simulink model "NXPFRDMK64F"  (R2022a)
settings: Solver=FixedStepAuto  StartTime=0.0  StopTime=60  FixedStep=1e-3  RelTol=1e-3  EnableMultiTasking=on
undefined symbols (not defined in the file): A0, A1, ARPtest, ATRsense, D0, D1, D10, D11, D12, D13, D2, D3, D4, D5, D6, D7, D8, D9, LRLtest, PTA0, PTA1, PTA2, PTB2, PTB23, PTB3, PTB9, PTC16, PTC17, PTC2, PTC3, PTC4, PTD0, PTD1, PTD2, PTD3, pulsewtest, URLtest, VENTsense, VRPtest
libraries: frdmk64flib x20, simulink x2, etargetslib x2
settings Model: ExtModeTrigDuration=5  Creator=patri  LastModifiedBy=David
settings OptimizationCC: EnhancedBackFolding=on  PassReuseOutputArgsAs=Individual arguments  ZeroExternalMemoryAtStartup=off  ZeroInternalMemoryAtStartup=off  MaxStackSize=64  OptimizeBlockOrder=speed  DifferentSizesBufferReuse=on  OptimizationCustomize=off  EfficientTunableParamExpr=on
settings DebuggingCC: ParameterTunabilityLossMsg=error
settings HardwareCC: ProdBitPerPointer=32  ProdBitPerSizeT=32  ProdBitPerPtrDiffT=32  ProdLargestAtomicInteger=Long  ProdLargestAtomicFloat=Double  ProdWordSize=32  ProdHWDeviceType=ARM Compatible->ARM Cortex
settings SFSimCC: MATLABDynamicMemAlloc=off
settings RTWCC: SystemTargetFile=ert.tlc  HardwareBoard=NXP FRDM-K64F  TLCOptions="-aInlineSetEventsForThisBaseRateFcn=TLC_FALSE -aSuppressMultiTaskScheduler=TLC_FALSE  -aRateBasedStepFcn=0"  TemplateMakefile=ert_default_tmf  Toolchain=GNU Tools for ARM Embedded Processors
settings CodeAppCC: ForceParamTrailComments=on  IgnoreCustomStorageClasses=off  OperatorAnnotations=on  SimulinkDataObjDesc=on  SFDataObjDesc=on  InsertBlockDesc=on
settings ERTTargetCC: ExtModeTransport=4  ExtModeMexFile=sendToCommService

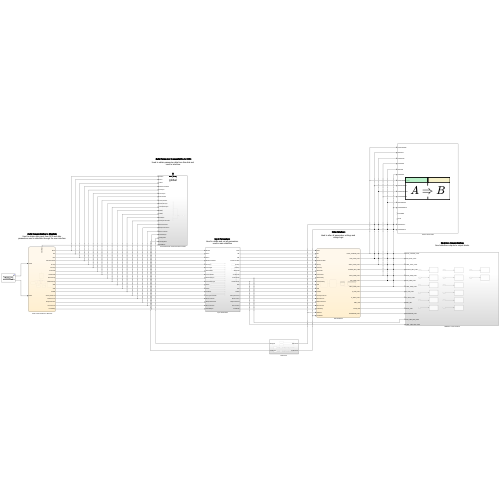
[thumbnail: Simulink's stored preview of the top-level diagram]
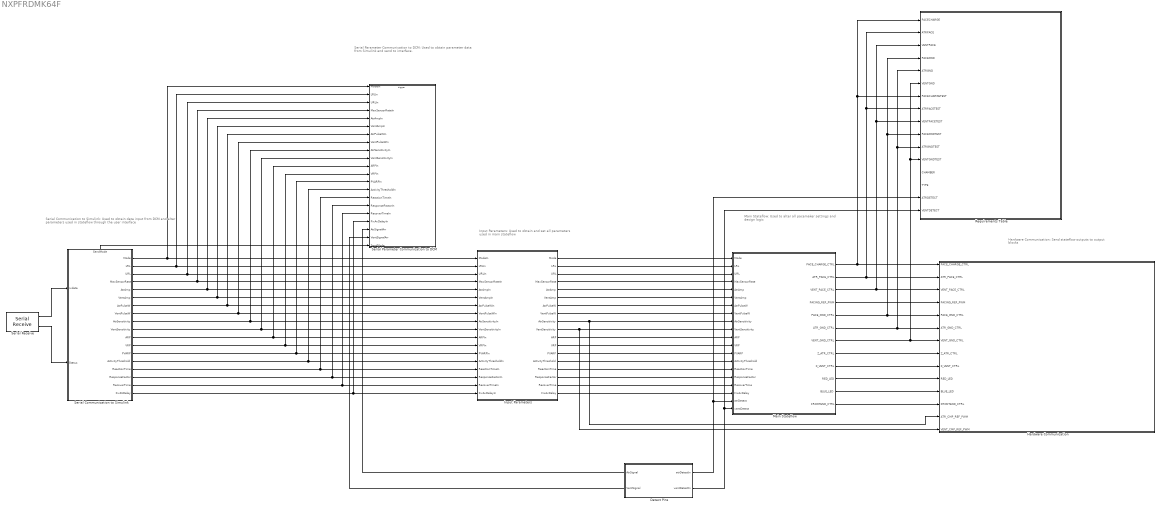
== system NXPFRDMK64F ==
  note: Input Parameters:
      | Used to obtain and set all parameters
      | used in main stateflow
  note: Main Stateflow:
      | Used to alter all pacemaker settings and
      | design logic
  note: Hardware Communication:
      | Send stateflow outputs to output blocks
  note: Serial Communication to Simulink:
      | Used to obtain data input from DCM and alter
      | parameters used in stateflow through the user interface
  note: Serial Parameter Communication to DCM:
      | Used to obtain parameter data from Simulink and
      | send to interface.
  Detect Pins : Subsystem
      settings: PortSchema="{\"entries\":[{\"content\":{\"sides\":[{\"content\":{\"connectorIds\":[\"Out3\",\"Out4\"]},\"type\":\"ConnectorPlacement.EquallySpacedRectSide\",\"uuid\":\"22ae5160-7907-4e02-9170-83912aa0621b\"},{\"content\":{\"connectorIds\":[\"Out1\",\"Out2\"],\"side\":\"RIGHT\"},\"type\":\"ConnectorPlacement.EquallySpacedRectSide\",\"uuid\":\"4a288593-63c5-4fb6-8cc6-6c5672326909\"},{\"content\":{\"connectorIds\":[],\"side\":\"TOP\"},\"type\":\"ConnectorPlacement.EquallySpacedRectSide\",\"uuid\":\"225d709c-1657-4037-9f08-1b7c425ad473\"}]},\"type\":\"ConnectorPlacement.EquallySpacedConnector\",\"uuid\":\"4f29d97d-bf7f-4e6d-a194-73bc61128bb5\"}],\"packageUris\":[\"http://schema.mathworks.com/mf0/Connector/R2020b\"],\"version\":\"1.0\"}"
  Hardware Communication : Subsystem
  Input Parameters : Subsystem
  Main Stateflow : Stateflow chart  TreatAsAtomicUnit=on
  Requirements Table : Requirements Table  TreatAsAtomicUnit=on
  Serial Communication to Simulink : Stateflow chart  TreatAsAtomicUnit=on
      settings: PortSchema="{\"entries\":[{\"content\":{\"sides\":[{\"content\":{\"connectorIds\":[\"In1\",\"In2\"]},\"type\":\"ConnectorPlacement.EquallySpacedRectSide\",\"uuid\":\"59d5f214-816c-4a61-90ca-5ecc2aac6342\"},{\"content\":{\"connectorIds\":[\"Out1\",\"Out2\",\"Out3\",\"Out4\",\"Out5\",\"Out6\",\"Out7\",\"Out8\",\"Out9\",\"Out10\",\"Out11\",\"Out12\",\"Out13\",\"Out14\",\"Out15\",\"Out16\",\"Out17\",\"Out18\"],\"side\":\"RIGHT\"},\"type\":\"ConnectorPlacement.EquallySpacedRectSide\",\"uuid\":\"caa3dc8d-9426-4e4b-b542-59ffb9e9ff55\"},{\"content\":{\"connectorIds\":[\"Out19\"],\"side\":\"TOP\"},\"type\":\"ConnectorPlacement.EquallySpacedRectSide\",\"uuid\":\"7c0b9c62-6555-43d5-acbe-ad9d7bd12e4a\"}]},\"type\":\"ConnectorPlacement.EquallySpacedConnector\",\"uuid\":\"af3c612b-0d58-4e05-b024-fac367dc3217\"}],\"packageUris\":[\"http://schema.mathworks.com/mf0/Connector/R2020b\"],\"version\":\"1.0\"}"
  Serial Parameter Communication to DCM : Subsystem  TreatAsAtomicUnit=on
  Serial Receive : frdmk64flib/Serial Receive  SCIModule=0  Baudrate=uint32(9600)  Parity=None  StopBits=1  HardwareFlowControl=None  ByteOrder=LittleEndian  DataType=uint8  DataLength=20  BlockingMode=off  OutputStatus=on  SampleTime=-1
  wires:
  Main Stateflow/1(PACE_CHARGE_CTRL) -> Requirements Table/1(PACECHARGE), Requirements Table/7(PACECHARGETEST), Hardware Communication/1(PACE_CHARGE_CTRL)
  Main Stateflow/3(VENT_PACE_CTRL) -> Requirements Table/3(VENTPACE), Requirements Table/9(VENTPACETEST), Hardware Communication/3(VENT_PACE_CTRL)
  Main Stateflow/4(PACING_REF_PWM) -> Hardware Communication/4(PACING_REF_PWM)
  Main Stateflow/5(PACE_GND_CTRL) -> Requirements Table/4(PACEGND), Requirements Table/10(PACEGNDTEST), Hardware Communication/5(PACE_GND_CTRL)
  Main Stateflow/8(Z_ATR_CTRL) -> Hardware Communication/8("Z_ATR_CTRL ")
  Main Stateflow/9(Z_VENT_CTRL) -> Hardware Communication/9(Z_VENT_CTRL)
  Main Stateflow/11(BLUE_LED) -> Hardware Communication/11(BLUE_LED)
  Main Stateflow/10(RED_LED) -> Hardware Communication/10(RED_LED)
  Main Stateflow/6(ATR_GND_CTRL) -> Requirements Table/5(ATRGND), Requirements Table/11(ATRGNDTEST), Hardware Communication/6(ATR_GND_CTRL)
  Main Stateflow/2(ATR_PACE_CTRL) -> Requirements Table/2(ATRPACE), Requirements Table/8(ATRPACETEST), Hardware Communication/2(ATR_PACE_CTRL)
  Main Stateflow/12(FRONTEND_CTRL) -> Hardware Communication/12(FRONTEND_CTRL)
  Detect Pins/2(ventDetectIn) -> Requirements Table/16(VENTDETECT), Main Stateflow/20(ventDetect)
  Serial Receive/1 -> Serial Communication to Simulink/1(rxdata)
  Serial Receive/2 -> Serial Communication to Simulink/2(Status)
  Main Stateflow/7(VENT_GND_CTRL) -> Requirements Table/6(VENTGND), Requirements Table/12(VENTGNDTEST), Hardware Communication/7(VENT_GND_CTRL)
  Detect Pins/1(atrDetectIn) -> Requirements Table/15(ATRDETECT), Main Stateflow/19(atrDetect)
  Serial Communication to Simulink/1(Mode) -> Serial Parameter Communication to DCM/1(ModeIn), Input Parameters/1(ModeIn)
  Serial Communication to Simulink/2(LRL) -> Serial Parameter Communication to DCM/2(LRLIn), Input Parameters/2(LRLIn)
  Serial Communication to Simulink/3(URL) -> Serial Parameter Communication to DCM/3(URLIn), Input Parameters/3(URLIn)
  Serial Communication to Simulink/4(MaxSensorRate) -> Serial Parameter Communication to DCM/4(MaxSensorRateIn), Input Parameters/4(MaxSensorRateIn)
  Serial Communication to Simulink/5(AtrAmp) -> Serial Parameter Communication to DCM/5(AtrAmpIn), Input Parameters/5(AtrAmpIn)
  Serial Communication to Simulink/7(AtrPulseW) -> Serial Parameter Communication to DCM/7(AtrPulseWIn), Input Parameters/7(AtrPulseWIn)
  Serial Communication to Simulink/6(VentAmp) -> Serial Parameter Communication to DCM/6(VentAmpIn), Input Parameters/6(VentAmpIn)
  Serial Communication to Simulink/8(VentPulseW) -> Serial Parameter Communication to DCM/8(VentPulseWIn), Input Parameters/8(VentPulseWIn)
  Serial Communication to Simulink/10(VentSensitivity) -> Serial Parameter Communication to DCM/10(VentSensitivityIn), Input Parameters/10(VentSensitivityIn)
  Serial Communication to Simulink/11(ARP) -> Serial Parameter Communication to DCM/11(ARPIn), Input Parameters/11(ARPIn)
  Serial Communication to Simulink/9(AtrSensitivity) -> Serial Parameter Communication to DCM/9(AtrSensitivityIn), Input Parameters/9(AtrSensitivityIn)
  Serial Communication to Simulink/12(VRP) -> Serial Parameter Communication to DCM/12(VRPIn), Input Parameters/12(VRPIn)
  Serial Communication to Simulink/13(PVARP) -> Serial Parameter Communication to DCM/13(PVARPIn), Input Parameters/13(PVARPIn)
  Serial Communication to Simulink/14(ActivityThreshold) -> Serial Parameter Communication to DCM/14(ActivityThresholdIn), Input Parameters/14(ActivityThresholdIn)
  Serial Communication to Simulink/15(ReactionTime) -> Serial Parameter Communication to DCM/15(ReactionTimeIn), Input Parameters/15(ReactionTimeIn)
  Serial Communication to Simulink/16(ResponseFactor) -> Serial Parameter Communication to DCM/16(ResponseFactorIn), Input Parameters/16(ResponseFactorIn)
  Serial Communication to Simulink/17(RecoverTime) -> Serial Parameter Communication to DCM/17(RecoverTimeIn), Input Parameters/17(RecoverTimeIn)
  Serial Communication to Simulink/18(FixAVDelay) -> Serial Parameter Communication to DCM/18(FixAvDelayIn), Input Parameters/18(FixAvDelayIn)
  Detect Pins/4(VentSignal) -> Serial Parameter Communication to DCM/20(VentSignalArr)
  Detect Pins/3(AtrSignal) -> Serial Parameter Communication to DCM/19(AtrSignalArr)
  Input Parameters/1(Mode) -> Main Stateflow/1(Mode)
  Input Parameters/2(LRL) -> Main Stateflow/2(LRL)
  Input Parameters/3(URL) -> Main Stateflow/3(URL)
  Input Parameters/4(MaxSensorRate) -> Main Stateflow/4(MaxSensorRate)
  Input Parameters/5(AtrAmp) -> Main Stateflow/5(AtrAmp)
  Input Parameters/6(VentAmp) -> Main Stateflow/6(VentAmp)
  Input Parameters/7(AtrPulseW) -> Main Stateflow/7(AtrPulseW)
  Input Parameters/8(VentPulseW) -> Main Stateflow/8(VentPulseW)
  Input Parameters/9(AtrSensitivity) -> Hardware Communication/13(ATR_CMP_REF_PWM), Main Stateflow/9(AtrSensitivity)
  Input Parameters/10(VentSensitivity) -> Hardware Communication/14(VENT_CMP_REF_PWM), Main Stateflow/10(VentSensitivity)
  Input Parameters/11(ARP) -> Main Stateflow/11(ARP)
  Input Parameters/14(ActivityThreshold) -> Main Stateflow/14(ActivityThreshold)
  Input Parameters/13(PVARP) -> Main Stateflow/13(PVARP)
  Input Parameters/12(VRP) -> Main Stateflow/12(VRP)
  Input Parameters/15(ReactionTime) -> Main Stateflow/15(ReactionTime)
  Input Parameters/16(ResponseFactor) -> Main Stateflow/16(ResponseFactor)
  Input Parameters/17(RecoverTime) -> Main Stateflow/17(RecoverTime)
  Input Parameters/18(FixAvDelay) -> Main Stateflow/18(FixAvDelay)
  Serial Communication to Simulink/19(SendMode) -> Serial Parameter Communication to DCM/21(SendMode)

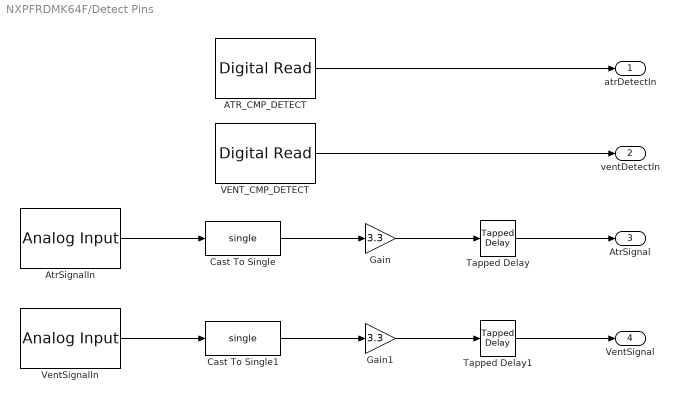
== system NXPFRDMK64F/Detect Pins ==
  ATR_CMP_DETECT : frdmk64flib/Digital Read  Whichpin=PTC16 (D0)  SampleTime=-1
  AtrSignalIn : frdmk64flib/Analog Input  Whichpin=PTB2 (A0)  SampleTime=-1
  Cast To Single : DataTypeConversion  OutDataTypeStr=single  SaturateOnIntegerOverflow=off  RndMeth=Floor
  Cast To Single1 : DataTypeConversion  OutDataTypeStr=single  SaturateOnIntegerOverflow=off  RndMeth=Floor
  Gain : Gain  Gain=3.3
  Gain1 : Gain  Gain=3.3
  Tapped Delay : simulink/Discrete/Tapped Delay  vinit=0.0  samptime=0.002  NumDelays=9  DelayOrder=Oldest  includeCurrent=off
  Tapped Delay1 : simulink/Discrete/Tapped Delay  vinit=0.0  samptime=0.002  NumDelays=9  DelayOrder=Oldest  includeCurrent=off
  VENT_CMP_DETECT : frdmk64flib/Digital Read  Whichpin=PTC17 (D1)  SampleTime=-1
  VentSignalIn : frdmk64flib/Analog Input  Whichpin=PTB3 (A1)  SampleTime=-1
  atrDetectIn : Outport
  ventDetectIn : Outport  Port=2
  AtrSignal : Outport  Port=3
  VentSignal : Outport  Port=4
  wires:
  VENT_CMP_DETECT/1 -> ventDetectIn/1
  ATR_CMP_DETECT/1 -> atrDetectIn/1
  AtrSignalIn/1 -> Cast To Single/1
  Cast To Single/1 -> Gain/1
  Gain/1 -> Tapped Delay/1
  Tapped Delay/1 -> AtrSignal/1
  Gain1/1 -> Tapped Delay1/1
  Cast To Single1/1 -> Gain1/1
  Tapped Delay1/1 -> VentSignal/1
  VentSignalIn/1 -> Cast To Single1/1

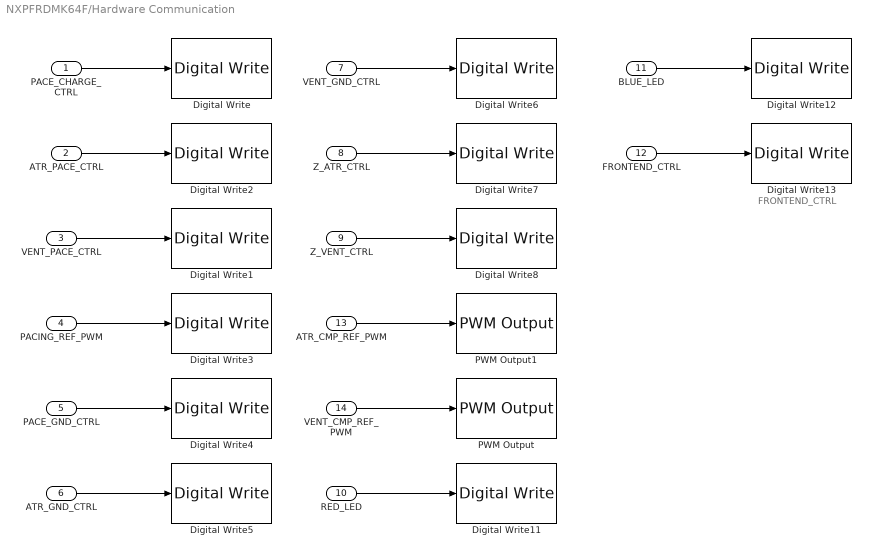
== system NXPFRDMK64F/Hardware Communication ==
  note: FRONTEND_CTRL
  PACE_CHARGE_CTRL : Inport
  ATR_PACE_CTRL : Inport  Port=2
  VENT_PACE_CTRL : Inport  Port=3
  PACING_REF_PWM : Inport  Port=4
  PACE_GND_CTRL : Inport  Port=5
  ATR_GND_CTRL : Inport  Port=6
  VENT_GND_CTRL : Inport  Port=7
  "Z_ATR_CTRL " : Inport  Port=8
  Z_VENT_CTRL : Inport  Port=9
  RED_LED : Inport  Port=10
  BLUE_LED : Inport  Port=11
  FRONTEND_CTRL : Inport  Port=12
  ATR_CMP_REF_PWM : Inport  Port=13
  VENT_CMP_REF_PWM : Inport  Port=14
  Digital Write : frdmk64flib/Digital Write  Whichpin=PTB9 (D2)
  Digital Write1 : frdmk64flib/Digital Write  Whichpin=PTC4 (D9)
  Digital Write11 : frdmk64flib/Digital Write  Whichpin=RED_LED
  Digital Write12 : frdmk64flib/Digital Write  Whichpin=BLUE_LED
  Digital Write13 : frdmk64flib/Digital Write  Whichpin=PTD1 (D13)
  Digital Write2 : frdmk64flib/Digital Write  Whichpin=PTA0 (D8)
  Digital Write3 : frdmk64flib/Digital Write  Whichpin=PTA2 (D5)
  Digital Write4 : frdmk64flib/Digital Write  Whichpin=PTD0 (D10)
  Digital Write5 : frdmk64flib/Digital Write  Whichpin=PTD2 (D11)
  Digital Write6 : frdmk64flib/Digital Write  Whichpin=PTD3 (D12)
  Digital Write7 : frdmk64flib/Digital Write  Whichpin=PTB23 (D4)
  Digital Write8 : frdmk64flib/Digital Write  Whichpin=PTC3 (D7)
  PWM Output : frdmk64flib/PWM Output  Whichpin=PTA1 (D3)  InitialFrequency=2000  InitialDutyCycle=0
  PWM Output1 : frdmk64flib/PWM Output  Whichpin=PTC2 (D6)  InitialFrequency=2000  InitialDutyCycle=0
  wires:
  "Z_ATR_CTRL "/1 -> Digital Write7/1
  ATR_CMP_REF_PWM/1 -> PWM Output1/1
  Z_VENT_CTRL/1 -> Digital Write8/1
  VENT_CMP_REF_PWM/1 -> PWM Output/1
  BLUE_LED/1 -> Digital Write12/1
  PACE_CHARGE_CTRL/1 -> Digital Write/1
  RED_LED/1 -> Digital Write11/1
  ATR_PACE_CTRL/1 -> Digital Write2/1
  VENT_PACE_CTRL/1 -> Digital Write1/1
  PACING_REF_PWM/1 -> Digital Write3/1
  PACE_GND_CTRL/1 -> Digital Write4/1
  ATR_GND_CTRL/1 -> Digital Write5/1
  VENT_GND_CTRL/1 -> Digital Write6/1
  FRONTEND_CTRL/1 -> Digital Write13/1

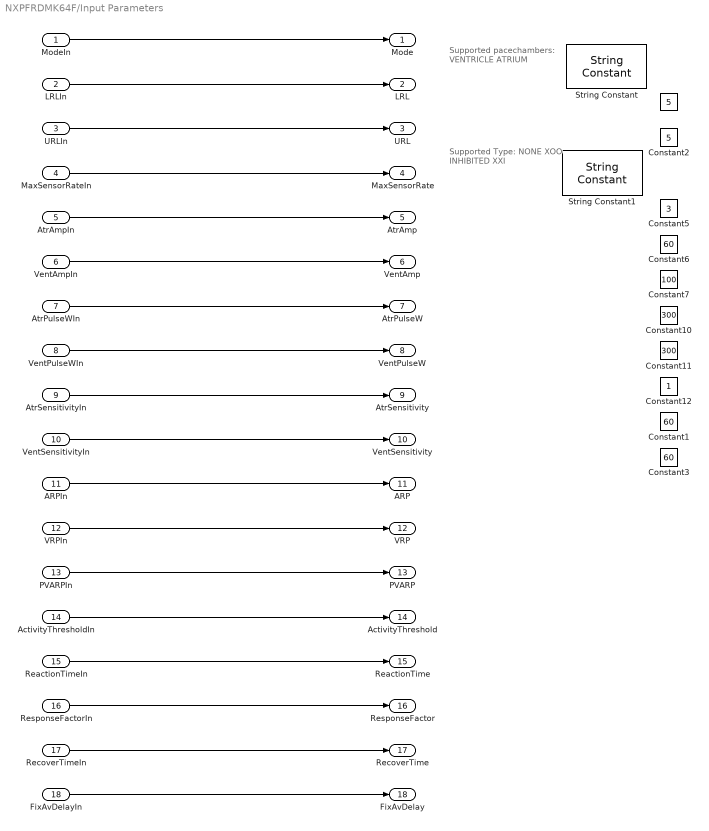
== system NXPFRDMK64F/Input Parameters ==
  note: Supported pacechambers:
      | VENTRICLE
      | ATRIUM
  note: Supported Type:
      | NONE XOO
      | INHIBITED XXI
  ModeIn : Inport
  LRLIn : Inport  Port=2
  URLIn : Inport  Port=3
  MaxSensorRateIn : Inport  Port=4
  AtrAmpIn : Inport  Port=5
  VentAmpIn : Inport  Port=6
  AtrPulseWIn : Inport  Port=7
  VentPulseWIn : Inport  Port=8
  AtrSensitivityIn : Inport  Port=9
  VentSensitivityIn : Inport  Port=10
  ARPIn : Inport  Port=11
  VRPIn : Inport  Port=12
  PVARPIn : Inport  Port=13
  ActivityThresholdIn : Inport  Port=14
  ReactionTimeIn : Inport  Port=15
  ResponseFactorIn : Inport  Port=16
  RecoverTimeIn : Inport  Port=17
  FixAvDelayIn : Inport  Port=18
  " " : Constant  Value=5
  Constant1 : Constant  Value=60
  Constant10 : Constant  Value=300
  Constant11 : Constant  Value=300
  Constant12 : Constant
  Constant2 : Constant  Value=5
  Constant3 : Constant  Value=60
  Constant5 : Constant  Value=3
  Constant6 : Constant  Value=60
  Constant7 : Constant  Value=100
  String Constant : StringConstant  String="\"ATRIUM\""
  String Constant1 : StringConstant  String="\"INHIBITED\""
  Mode : Outport
  LRL : Outport  Port=2
  URL : Outport  Port=3
  MaxSensorRate : Outport  Port=4
  AtrAmp : Outport  Port=5
  VentAmp : Outport  Port=6
  AtrPulseW : Outport  Port=7
  VentPulseW : Outport  Port=8
  AtrSensitivity : Outport  Port=9
  VentSensitivity : Outport  Port=10
  ARP : Outport  Port=11
  VRP : Outport  Port=12
  PVARP : Outport  Port=13
  ActivityThreshold : Outport  Port=14
  ReactionTime : Outport  Port=15
  ResponseFactor : Outport  Port=16
  RecoverTime : Outport  Port=17
  FixAvDelay : Outport  Port=18
  wires:
  ModeIn/1 -> Mode/1
  LRLIn/1 -> LRL/1
  URLIn/1 -> URL/1
  MaxSensorRateIn/1 -> MaxSensorRate/1
  AtrAmpIn/1 -> AtrAmp/1
  VentAmpIn/1 -> VentAmp/1
  AtrPulseWIn/1 -> AtrPulseW/1
  VentPulseWIn/1 -> VentPulseW/1
  AtrSensitivityIn/1 -> AtrSensitivity/1
  VentSensitivityIn/1 -> VentSensitivity/1
  ARPIn/1 -> ARP/1
  VRPIn/1 -> VRP/1
  PVARPIn/1 -> PVARP/1
  ActivityThresholdIn/1 -> ActivityThreshold/1
  ReactionTimeIn/1 -> ReactionTime/1
  ResponseFactorIn/1 -> ResponseFactor/1
  RecoverTimeIn/1 -> RecoverTime/1
  FixAvDelayIn/1 -> FixAvDelay/1

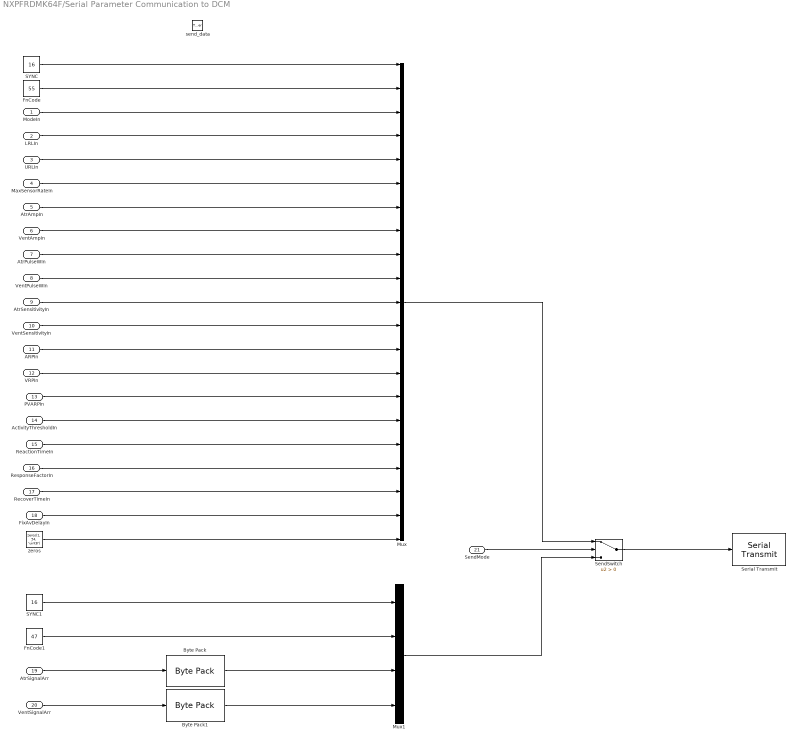
== system NXPFRDMK64F/Serial Parameter Communication to DCM ==
  ModeIn : Inport
  LRLIn : Inport  Port=2
  URLIn : Inport  Port=3
  MaxSensorRateIn : Inport  Port=4
  AtrAmpIn : Inport  Port=5
  VentAmpIn : Inport  Port=6
  AtrPulseWIn : Inport  Port=7
  VentPulseWIn : Inport  Port=8
  AtrSensitivityIn : Inport  Port=9
  VentSensitivityIn : Inport  Port=10
  ARPIn : Inport  Port=11
  VRPIn : Inport  Port=12
  PVARPIn : Inport  Port=13
  ActivityThresholdIn : Inport  Port=14
  ReactionTimeIn : Inport  Port=15
  ResponseFactorIn : Inport  Port=16
  RecoverTimeIn : Inport  Port=17
  FixAvDelayIn : Inport  Port=18
  AtrSignalArr : Inport  Port=19  OutDataTypeStr=single
  VentSignalArr : Inport  Port=20  OutDataTypeStr=single
  SendMode : Inport  Port=21
  send_data : TriggerPort  TriggerType=function-call  IsSimulinkFunction=on  FunctionName=send_data  VariantControl=(inherit)
  Byte Pack : etargetslib/Byte Pack  datatypes={'single'}  byteAlign=1
  Byte Pack1 : etargetslib/Byte Pack  datatypes={'single'}  byteAlign=1
  FnCode : Constant  Value=55  OutDataTypeStr=uint8
  FnCode1 : Constant  Value=47  OutDataTypeStr=uint8
  Mux : Mux  Inputs=21
  Mux1 : Mux
  SYNC : Constant  Value=16  OutDataTypeStr=uint8
  SYNC1 : Constant  Value=16  OutDataTypeStr=uint8
  SendSwitch : Switch  Criteria=u2 > Threshold  SaturateOnIntegerOverflow=off  InputSameDT=off
  Serial Transmit : frdmk64flib/Serial Transmit  SCIModule=0  Baudrate=uint32(9600)  Parity=None  StopBits=1  HardwareFlowControl=None  ByteOrder=LittleEndian  BlockingMode=on  OutputStatus=off
  zeros : Constant  Value=zeros(1, 54, 'uint8')
  wires:
  Mux1/1 -> SendSwitch/3
  FnCode1/1 -> Mux1/2
  Byte Pack1/1 -> Mux1/4
  Byte Pack/1 -> Mux1/3
  SendSwitch/1 -> Serial Transmit/1
  VentPulseWIn/1 -> Mux/10
  SendMode/1 -> SendSwitch/2
  FnCode/1 -> Mux/2
  ARPIn/1 -> Mux/13
  VRPIn/1 -> Mux/14
  VentSignalArr/1 -> Byte Pack1/1
  SYNC/1 -> Mux/1
  ReactionTimeIn/1 -> Mux/17
  AtrSignalArr/1 -> Byte Pack/1
  URLIn/1 -> Mux/5
  AtrAmpIn/1 -> Mux/7
  ActivityThresholdIn/1 -> Mux/16
  Mux/1 -> SendSwitch/1
  AtrSensitivityIn/1 -> Mux/11
  VentAmpIn/1 -> Mux/8
  zeros/1 -> Mux/21
  AtrPulseWIn/1 -> Mux/9
  ModeIn/1 -> Mux/3
  RecoverTimeIn/1 -> Mux/19
  ResponseFactorIn/1 -> Mux/18
  LRLIn/1 -> Mux/4
  PVARPIn/1 -> Mux/15
  SYNC1/1 -> Mux1/1
  MaxSensorRateIn/1 -> Mux/6
  FixAvDelayIn/1 -> Mux/20
  VentSensitivityIn/1 -> Mux/12

== stateflow chart NXPFRDMK64F/Requirements Table ==
  (default) -> (junction 1073743439)
  (junction 1073743439) -> (junction 1073743440) : {
      | % SF_REQ_REV_07
      | }
  (junction 1073743440) -> (junction 1073743442) : {
      | % HEADER_ASSIGNMENTS
      |
      | }
  (junction 1073743442) -> (junction 1073743444) : {
      | % START_A_4
      | }
  (junction 1073743444) -> (junction 1073743446) : {
      | }
  (junction 1073743446) -> (junction 1073743448)
  (junction 1073743448) -> (junction 1073743450) : {
      | }
  (junction 1073743450) -> (junction 1073743452) : {
      | % END_A_4
      | }
  (junction 1073743452) -> (junction 1073743454) : {
      | % START_R_1
      | }
  (junction 1073743454) -> (junction 1073743456) : {
      | }
  (junction 1073743456) -> (junction 1073743458)
  (junction 1073743458) -> (junction 1073743460) [order 1] : [(((TYPE) == ("NONE"))) && (((CHAMBER) == ("ATRIUM")))]
  (junction 1073743458) -> (junction 1073743466) [order 2]
  (junction 1073743460) -> (junction 1073743462) : {
      | reqtable_postcondition((((PACECHARGETEST) == (0))) && (((ATRPACETEST) == (1))) && (((VENTPACETEST) == (0))) && (((PACEGNDTEST) == (1))) && (((ATRGNDTEST) == (0))) && (((VENTGNDTEST) == (0))), 'R:1');
      |
      |
      | }
  (junction 1073743462) -> (junction 1073743464) : {
      | }
  (junction 1073743464) -> (junction 1073743466)
  (junction 1073743466) -> (junction 1073743468)
  (junction 1073743468) -> (junction 1073743470) : {
      | % END_R_1
      | }
  (junction 1073743470) -> (junction 1073743472) : {
      | % START_R_10
      | }
  (junction 1073743472) -> (junction 1073743474) : {
      | }
  (junction 1073743474) -> (junction 1073743476)
  (junction 1073743476) -> (junction 1073743478) [order 1] : [(((TYPE) == ("NONE"))) && (((CHAMBER) == ("ATRIUM"))) && (((PACECHARGE) == (0))) && (((ATRPACE) == (1))) && (((VENTPACE) == (0))) && (((PACEGND) == (1))) && (((ATRGND) == (0))) && (((VENTGND) == (0)))]
  (junction 1073743476) -> (junction 1073743484) [order 2]
  (junction 1073743478) -> (junction 1073743480) : {
      | reqtable_postcondition((((PACECHARGETEST) == (1))) && (((ATRPACETEST) == (0))) && (((VENTPACETEST) == (0))) && (((PACEGNDTEST) == (0))) && (((ATRGNDTEST) == (1))) && (((VENTGNDTEST) == (0))), 'R:2');
      |
      |
      | }
  (junction 1073743480) -> (junction 1073743482) : {
      | }
  (junction 1073743482) -> (junction 1073743484)
  (junction 1073743484) -> (junction 1073743486)
  (junction 1073743486) -> (junction 1073743488) : {
      | % END_R_10
      | }
  (junction 1073743488) -> (junction 1073743490) : {
      | % START_R_7
      | }
  (junction 1073743490) -> (junction 1073743492) : {
      | }
  (junction 1073743492) -> (junction 1073743494)
  (junction 1073743494) -> (junction 1073743496) [order 1] : [(((TYPE) == ("NONE"))) && (((CHAMBER) == ("VENTRICLE")))]
  (junction 1073743494) -> (junction 1073743502) [order 2]
  (junction 1073743496) -> (junction 1073743498) : {
      | reqtable_postcondition((((PACECHARGETEST) == (0))) && (((ATRPACETEST) == (0))) && (((VENTPACETEST) == (1))) && (((PACEGNDTEST) == (1))) && (((ATRGNDTEST) == (0))) && (((VENTGNDTEST) == (0))), 'R:3');
      |
      |
      | }
  (junction 1073743498) -> (junction 1073743500) : {
      | }
  (junction 1073743500) -> (junction 1073743502)
  (junction 1073743502) -> (junction 1073743504)
  (junction 1073743504) -> (junction 1073743506) : {
      | % END_R_7
      | }
  (junction 1073743506) -> (junction 1073743508) : {
      | % START_R_13
      | }
  (junction 1073743508) -> (junction 1073743510) : {
      | }
  (junction 1073743510) -> (junction 1073743512)
  (junction 1073743512) -> (junction 1073743514) [order 1] : [(((TYPE) == ("NONE"))) && (((CHAMBER) == ("VENTRICLE"))) && (((PACECHARGE) == (0))) && (((ATRPACE) == (0))) && (((VENTPACE) == (1))) && (((PACEGND) == (1))) && (((ATRGND) == (0))) && (((VENTGND) == (0)))]
  (junction 1073743512) -> (junction 1073743520) [order 2]
  (junction 1073743514) -> (junction 1073743516) : {
      | reqtable_postcondition((((PACECHARGETEST) == (1))) && (((ATRPACETEST) == (0))) && (((VENTPACETEST) == (0))) && (((PACEGNDTEST) == (0))) && (((ATRGNDTEST) == (0))) && (((VENTGNDTEST) == (1))), 'R:4');
      |
      |
      | }
  (junction 1073743516) -> (junction 1073743518) : {
      | }
  (junction 1073743518) -> (junction 1073743520)
  (junction 1073743520) -> (junction 1073743522)
  (junction 1073743522) -> (junction 1073743524) : {
      | % END_R_13
      | }
  (junction 1073743524) -> (junction 1073743526) : {
      | % START_R_16
      | }
  (junction 1073743526) -> (junction 1073743528) : {
      | }
  (junction 1073743528) -> (junction 1073743530)
  (junction 1073743530) -> (junction 1073743532) [order 1] : [(((TYPE) == ("INHIBITED"))) && (((ATRDETECT) == (1))) && (((CHAMBER) == ("ATRIUM")))]
  (junction 1073743530) -> (junction 1073743538) [order 2]
  (junction 1073743532) -> (junction 1073743534) : {
      | reqtable_postcondition((((PACECHARGETEST) == (1))) && (((ATRPACETEST) == (0))) && (((VENTPACETEST) == (0))) && (((PACEGNDTEST) == (0))) && (((ATRGNDTEST) == (0))) && (((VENTGNDTEST) == (0))), 'R:5');
      |
      |
      | }
  (junction 1073743534) -> (junction 1073743536) : {
      | }
  (junction 1073743536) -> (junction 1073743538)
  (junction 1073743538) -> (junction 1073743540)
  (junction 1073743540) -> (junction 1073743542) : {
      | % END_R_16
      | }
  (junction 1073743542) -> (junction 1073743544) : {
      | % START_R_28
      | }
  (junction 1073743544) -> (junction 1073743546) : {
      | }
  (junction 1073743546) -> (junction 1073743548)
  (junction 1073743548) -> (junction 1073743550) [order 1] : [(((TYPE) == ("INHIBITED"))) && (((ATRDETECT) == (1))) && (((CHAMBER) == ("ATRIUM")))]
  (junction 1073743548) -> (junction 1073743556) [order 2]
  (junction 1073743550) -> (junction 1073743552) : {
      | reqtable_postcondition((((PACECHARGETEST) == (1))) && (((ATRPACETEST) == (0))) && (((VENTPACETEST) == (0))) && (((PACEGNDTEST) == (1))) && (((ATRGNDTEST) == (1))) && (((VENTGNDTEST) == (0))), 'R:6');
      |
      |
      | }
  (junction 1073743552) -> (junction 1073743554) : {
      | }
  (junction 1073743554) -> (junction 1073743556)
  (junction 1073743556) -> (junction 1073743558)
  (junction 1073743558) -> (junction 1073743560) : {
      | % END_R_28
      | }
  (junction 1073743560) -> (junction 1073743562) : {
      | % START_R_19
      | }
  (junction 1073743562) -> (junction 1073743564) : {
      | }
  (junction 1073743564) -> (junction 1073743566)
  (junction 1073743566) -> (junction 1073743568) [order 1] : [(((TYPE) == ("INHIBITIED"))) && (((ATRDETECT) == (0))) && (((CHAMBER) == ("ATRIUM")))]
  (junction 1073743566) -> (junction 1073743574) [order 2]
  (junction 1073743568) -> (junction 1073743570) : {
      | reqtable_postcondition((((PACECHARGETEST) == (0))) && (((ATRPACETEST) == (1))) && (((VENTPACETEST) == (0))) && (((PACEGNDTEST) == (1))) && (((ATRGNDTEST) == (0))) && (((VENTGNDTEST) == (0))), 'R:7');
      |
      |
      | }
  (junction 1073743570) -> (junction 1073743572) : {
      | }
  (junction 1073743572) -> (junction 1073743574)
  (junction 1073743574) -> (junction 1073743576)
  (junction 1073743576) -> (junction 1073743578) : {
      | % END_R_19
      | }
  (junction 1073743578) -> (junction 1073743580) : {
      | % START_R_22
      | }
  (junction 1073743580) -> (junction 1073743582) : {
      | }
  (junction 1073743582) -> (junction 1073743584)
  (junction 1073743584) -> (junction 1073743586) [order 1] : [(((TYPE) == ("INHIBITED"))) && (((VENTDETECT) == (1))) && (((CHAMBER) == ("VENTRICLE")))]
  (junction 1073743584) -> (junction 1073743592) [order 2]
  (junction 1073743586) -> (junction 1073743588) : {
      | reqtable_postcondition((((PACECHARGETEST) == (1))) && (((ATRPACETEST) == (0))) && (((VENTPACETEST) == (0))) && (((PACEGNDTEST) == (0))) && (((ATRGNDTEST) == (0))) && (((VENTGNDTEST) == (0))), 'R:8');
      |
      |
      | }
  (junction 1073743588) -> (junction 1073743590) : {
      | }
  (junction 1073743590) -> (junction 1073743592)
  (junction 1073743592) -> (junction 1073743594)
  (junction 1073743594) -> (junction 1073743596) : {
      | % END_R_22
      | }
  (junction 1073743596) -> (junction 1073743598) : {
      | % START_R_31
      | }
  (junction 1073743598) -> (junction 1073743600) : {
      | }
  (junction 1073743600) -> (junction 1073743602)
  (junction 1073743602) -> (junction 1073743604) [order 1] : [(((TYPE) == ("INHIBITED"))) && (((VENTDETECT) == (1))) && (((CHAMBER) == ("VENTRICLE")))]
  (junction 1073743602) -> (junction 1073743610) [order 2]
  (junction 1073743604) -> (junction 1073743606) : {
      | reqtable_postcondition((((PACECHARGETEST) == (1))) && (((ATRPACETEST) == (0))) && (((VENTPACETEST) == (0))) && (((PACEGNDTEST) == (1))) && (((ATRGNDTEST) == (0))) && (((VENTGNDTEST) == (1))), 'R:9');
      |
      |
      | }
  (junction 1073743606) -> (junction 1073743608) : {
      | }
  (junction 1073743608) -> (junction 1073743610)
  (junction 1073743610) -> (junction 1073743612)
  (junction 1073743612) -> (junction 1073743614) : {
      | % END_R_31
      | }
  (junction 1073743614) -> (junction 1073743616) : {
      | % START_R_25
      | }
  (junction 1073743616) -> (junction 1073743618) : {
      | }
  (junction 1073743618) -> (junction 1073743620)
  (junction 1073743620) -> (junction 1073743622) [order 1] : [(((TYPE) == ("INHIBITED"))) && (((VENTDETECT) == (0))) && (((CHAMBER) == ("VENTRICLE")))]
  (junction 1073743620) -> (junction 1073743628) [order 2]
  (junction 1073743622) -> (junction 1073743624) : {
      | reqtable_postcondition((((PACECHARGETEST) == (0))) && (((ATRPACETEST) == (0))) && (((VENTPACETEST) == (1))) && (((PACEGNDTEST) == (1))) && (((ATRGNDTEST) == (0))) && (((VENTGNDTEST) == (0))), 'R:10');
      |
      |
      | }
  (junction 1073743624) -> (junction 1073743626) : {
      | }
  (junction 1073743626) -> (junction 1073743628)
  (junction 1073743628) -> (junction 1073743630)
  (junction 1073743630) -> (junction 1073743632) : {
      | % END_R_25
      | }
  data: PACECHARGE input; ATRPACE input; VENTPACE input; PACEGND input; ATRGND input; VENTGND input; LRLtest parameter; pulsewtest parameter; VRPtest parameter; URLtest parameter; PACECHARGETEST input; ATRPACETEST input; VENTPACETEST input; PACEGNDTEST input; ATRGNDTEST input; VENTGNDTEST input; CHAMBER input; TYPE input; ATRDETECT input; VENTDETECT input; ATRsense parameter; VENTsense parameter; ARPtest parameter; data1 local; data2 local

== stateflow chart NXPFRDMK64F/Serial Communication to Simulink ==
  state Initialize
    %Set default values
    entry:
    Mode = 1;
    LRL = 60;
    URL = 120;
    AtrAmp = 50;
    VentAmp = 50;
    AtrPulseW = 1;
    VentPulseW = 1;
    ARP = 25;
    VRP = 32;
    PVARP = 25;
    FixAVDelay = 15;
    MaxSensorRate = 120;
    ReactionTime = 30;
    ResponseFactor = 8;
    RecoverTime = 5;
    AtrSensitivity = 25;
    VentSensitivity = 25;
    ActivityThreshold = 28;
  note: Mode Numbers:
      | 1 = AOO
      | 2 = VOO
      | 3 = AAI
      | 4 = VVI
      | 5 = AOOR
      | 6 = VOOR
      | 7 = AAIR
      | 8 = VVIR
  state StandBy
    %Wait for DCM communication
  state Echo
    %Send Simulink parameter data to DCM
    SendMode = 0;
    send_data();
  state SetParams
    entry:
    Mode = rxdata(3);
    LRL = rxdata(4);
    URL = rxdata(5);
    MaxSensorRate = rxdata(6);
    AtrAmp = rxdata(7);
    VentAmp = rxdata(8);
    AtrPulseW = rxdata(9);
    VentPulseW = rxdata(10);
    AtrSensitivity = rxdata(11);
    VentSensitivity = rxdata(12);
    ARP = rxdata(13);
    VRP = rxdata(14);
    PVARP = rxdata(15);
    ActivityThreshold = rxdata(16);
    ReactionTime = rxdata(17);
    ResponseFactor = rxdata(18);
    RecoverTime = rxdata(19);
    FixAVDelay = rxdata(20);
  state ECGStop
    %Stop Simulink ECG data to DCM
    SendMode = 0;
  state SendECG
    %Send Simulink ECG data to DCM
    SendMode = 1;
    send_data();
  (default) -> Initialize
  Initialize -> StandBy
  Echo -> StandBy
  SetParams -> StandBy
  SendECG -> StandBy
  ECGStop -> StandBy
  StandBy -> (junction 65) : [Status == 0]
  (junction 65) -> (junction 66) : [rxdata(1) == 16]
  (junction 66) -> Echo [order 4] : [rxdata(2) == 49]
  (junction 66) -> SetParams [order 1] : [rxdata(2) == 55]
  (junction 66) -> SendECG [order 2] : [rxdata(2) == 47]
  (junction 66) -> ECGStop [order 3] : [rxdata(2) == 62]
  data: Mode output uint8; LRL output uint8; URL output uint8; MaxSensorRate output uint8; AtrAmp output uint8; VentAmp output uint8; AtrPulseW output uint8; VentPulseW output uint8; AtrSensitivity output uint8; VentSensitivity output uint8; rxdata input; Status input; ARP output uint8; VRP output uint8; PVARP output uint8; ActivityThreshold output uint8; ReactionTime output uint8; ResponseFactor output uint8; RecoverTime output uint8; FixAVDelay output uint8; SendMode output

== stateflow chart NXPFRDMK64F/Main Stateflow ==
  note: SensingStateflow
      | Holds the logic for sensing heart activity and responding to it. The letter code is considered before branching deeper based on the chamber sensed
  state SetState
    if Mode == 1
    pacechamber == "ATRIUM";
    Type == "NONE";
    elseif Mode == 2
    pacechamber == "VENTRICLE";
    Type == "NONE";
    elseif Mode == 3
    pacechamber == "ATRIUM";
    Type == "INHIBITED";
    elseif Mode == 4
    pacechamber == "VENTRICLE";
    Type == "INHIBITED";
    elseif Mode == 5
    pacechamber == "ATRIUM";
    Type == "R_NONE";
    elseif Mode == 6
    pacechamber == "VENTRICLE";
    Type == "R_NONE";
    elseif Mode == 7
    pacechamber == "ATRIUM";
    Type == "R_INHIBITED";
    elseif Mode == 8
    pacechamber == "VENTRICLE";
    Type == "R_INHIBITED";
    end
  state Initialize
    FRONTEND_CTRL = true;
    %Reset LEDS
    RED_LED = false;
    BLUE_LED = false;
    Z_VENT_CTRL = false;
    Z_ATR_CTRL = false;
    % selecting correct initial pulse amplitude
    if pacechamber == "VENTRICLE"
    pulsew = VentPulseW;
    PulseAmp = VentAmp;
    else
    pulsew = AtrPulseW;
    PulseAmp = AtrAmp;
    end
    %Set default values
    PACING_REF_PWM = (PulseAmp/5);
    VENT_PACE_CTRL = false;
    ATR_PACE_CTRL = false;
    PACE_GND_CTRL = true;
    VENT_GND_CTRL = false;
    ATR_GND_CTRL = false;
    PACE_CHARGE_CTRL = true;
    DelayCarry = 0;
  note: PacingStateflow
      | Holds the logic for pacing each chamber.
  state Pace
    state AtriumPace
      ATR_PACE_CTRL = true;
      %LED to display state
      RED_LED = true;
    state ChargeC22_DischargeC21
      %Discharge C21
      %Ensure patient is never directly connect to PWM
      VENT_PACE_CTRL = false;
      ATR_PACE_CTRL = false;
      PACE_GND_CTRL = true;
      %Check for what chamber is to be paced
      if pacechamber == "ATRIUM"
      ATR_GND_CTRL = true;
      VENT_GND_CTRL = false;
      else
      ATR_GND_CTRL = false;
      VENT_GND_CTRL = true;
      end
      %Charge C22
      if pacechamber == "VENTRICLE"
      PACING_REF_PWM = (VentAmp/5);
      else
      PACING_REF_PWM = (AtrAmp/5);
      end
      PACE_CHARGE_CTRL = true;
      %LED "blinks" for each pace
      RED_LED = false;
      BLUE_LED = false;
      %Exit out to sense again
      send(endpace)
    state ClearSignal
      %Clear signal before pacing
      ATR_GND_CTRL = false;
      PACE_GND_CTRL = true;
      VENT_GND_CTRL = false;
      PACE_CHARGE_CTRL = false;
    state VentriclePace
      VENT_PACE_CTRL = true;
      %LED to display state
      BLUE_LED = true;
    AtriumPace -> ChargeC22_DischargeC21 : after(pulsew,msec)
        | {DelayCarry = pulsew}
    ClearSignal -> AtriumPace [order 1] : [pacechamber == "ATRIUM"]
    (default) -> ClearSignal
    ClearSignal -> VentriclePace [order 2] : [pacechamber == "VENTRICLE"]
    VentriclePace -> ChargeC22_DischargeC21 : after(pulsew,msec)
        | {DelayCarry = pulsew}
  state Sense
    note: Default exists to constantly check if the mode is the same or is changed for the next cycle.
    note: Loops back for sensed case in inhibited
    note: Loops back for sensed case in inhibited
    note: Ventricle modes
    note: Atrium modes
    state Atrium
      state None
        %Wait for a time then pace
        send(startpace)
      state Default
      state Pace
        send(startpace)
      state Inhibited
        %checks if the heart is already paced
        %Reset carry for the next cycle
        DelayCarry = 0;
        send(A_Loop)
      state Buffer
        %delay
        delaytest = DelayCarry;
      (default) -> Sense.Atrium.Default
      (junction 208) -> Sense.Atrium.None [order 1] : after(60000/LRL,msec)
          | [Type == "NONE"]
      Sense.Atrium.Default -> (junction 208)
      Sense.Atrium.Buffer -> Sense.Atrium.Pace [order 2] : after((60000/LRL)-DelayCarry,msec)
      (junction 208) -> Sense.Atrium.Buffer [order 2] : after(ARP,msec)
          |  [Type == "INHIBITED"]
          | {DelayCarry = DelayCarry+ARP}
      Sense.Atrium.Buffer -> Sense.Atrium.Inhibited [order 1] : [atrDetect]
    state Ventricle
      state None
        %Wait for a time then pace
        send(startpace)
      state Default
      state Pace
        send(startpace)
      state Inhibited
        %checks if the heart is already paced
        %Reset carry for the next cycle
        DelayCarry = 0;
        send(V_Loop)
      state Buffer
        %delay
        delaytest = DelayCarry;
      (default) -> Sense.Ventricle.Default
      (junction 222) -> Sense.Ventricle.None [order 1] : after(60000/LRL ,msec)
          | [Type  == "NONE"]
      Sense.Ventricle.Default -> (junction 222)
      Sense.Ventricle.Buffer -> Sense.Ventricle.Pace [order 2] : after((60000/LRL)-DelayCarry,msec)
      (junction 222) -> Sense.Ventricle.Buffer [order 2] : after(VRP,msec)
          |  [Type == "INHIBITED"]
          | {DelayCarry = DelayCarry+VRP}
      Sense.Ventricle.Buffer -> Sense.Ventricle.Inhibited [order 1] : [ventDetect]
    state Default
    (default) -> Sense.Default
    Atrium -> Sense.Default : A_Loop
    Ventricle -> Sense.Default : V_Loop
    Sense.Default -> Atrium [order 2] : [pacechamber=="ATRIUM"]
    Sense.Default -> Ventricle [order 1] : [pacechamber=="VENTRICLE"]
  (default) -> SetState
  Sense -> Pace : startpace
  SetState -> Initialize
  Initialize -> Sense
  Pace -> Sense : endpace
  data: Mode input; LRL input; URL input; MaxSensorRate input; PACE_CHARGE_CTRL output; ATR_PACE_CTRL output; VENT_PACE_CTRL output; PACING_REF_PWM output; PACE_GND_CTRL output; ATR_GND_CTRL output; VENT_GND_CTRL output; Z_ATR_CTRL output; Z_VENT_CTRL output; AtrAmp input; VentAmp input; AtrPulseW input; VentPulseW input; AtrSensitivity input; VentSensitivity input; RED_LED output; BLUE_LED output; PulseAmp local; ARP input; VRP input; PVARP input; ActivityThreshold input; ReactionTime input; ResponseFactor input; RecoverTime input; FixAvDelay input; atrDetect input; ventDetect input; DelayCarry local; FRONTEND_CTRL output; pacechamber local; Type local; pulsew local
  events: startpace local FUNCTION_CALL_EVENT; endpace local FUNCTION_CALL_EVENT; V_Loop local FUNCTION_CALL_EVENT; A_Loop local FUNCTION_CALL_EVENT
